simulink model "clik_inverse"  (R2022b)
settings: Solver=ode1  StartTime=0.0  StopTime=4  FixedStep=0.001  RelTol=1e-3
undefined symbols (not defined in the file or in its folder): DiscIntNeverNeededParam, q0, Tc
settings Model: Creator=Xp  LastModifiedBy=brigh
settings SolverCC: AlgebraicLoopSolver=TrustRegion
settings DataIOCC: LimitDataPoints=on  SaveFormat=Array  SignalLoggingSaveFormat=ModelDataLogs  ReturnWorkspaceOutputs=off
settings OptimizationCC: ExpressionDepthLimit=2147483647  InitFltsAndDblsToZero=on  LifeSpan=inf
settings DebuggingCC: SaveWithParameterizedLinksMsg=none  UnderspecifiedInitializationDetection=Classic  MergeDetectMultiDrivingBlocksExec=none  SolverPrmCheckMsg=warning  MultiTaskDSMMsg=warning  MultiTaskCondExecSysMsg=none  FcnCallInpInsideContextMsg=warning  UnconnectedInputMsg=warning  UnconnectedOutputMsg=warning  UnconnectedLineMsg=warning  StateNameClashWarn=warning  SFUnexpectedBacktrackingDiag=warning  SFNoUnconditionalDefaultTransitionDiag=warning  SFExecutionAtInitializationDiag=none  SFMachineParentedDataDiag=warning  ArithmeticOperatorsInVariantConditions=warning
settings HardwareCC: ProdBitPerPointer=32  ProdBitPerSizeT=32  ProdBitPerPtrDiffT=32  ProdLargestAtomicFloat=None  ProdIntDivRoundTo=Undefined  ProdEndianess=Unspecified  ProdWordSize=32  ProdHWDeviceType=32-bit Generic
settings ModelReferenceCC: EnableRefExpFcnMdlSchedulingChecks=on  PropagateSignalLabelsOutOfModel=off
settings SFSimCC: CustomCodeUndefinedFunction=UseInterfaceOnly
settings RTWCC: DLArmComputeVersion=19.05
settings CodeAppCC: StateflowObjectComments=on
settings GRTTargetCC: TargetLangStandard=C89/C90 (ANSI)  CombineOutputUpdateFcns=off  GRTInterface=on
settings ConfigComp: CovMetricSettings=dw  CovSaveCumulativeToWorkspaceVar=on  CovSaveSingleToWorkspaceVar=on

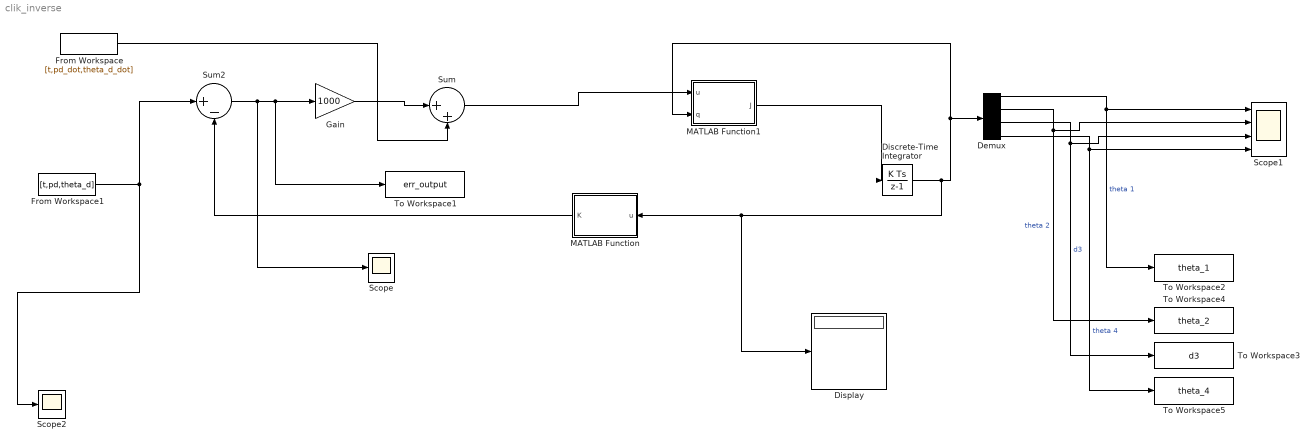
== system clik_inverse ==
  Demux : Demux
  Discrete-Time Integrator : DiscreteIntegrator  InitialCondition=q0  SampleTime=Tc  ICPrevOutput=DiscIntNeverNeededParam  ICPrevScaledInput=DiscIntNeverNeededParam
  Display : Display
  From Workspace : FromWorkspace  VariableName=[t,pd_dot,theta_d_dot]  SampleTime=Tc
  From Workspace1 : FromWorkspace  VariableName=[t,pd,theta_d]  SampleTime=Tc
  Gain : Gain  Gain=1000
  MATLAB Function : MATLAB Function  TreatAsAtomicUnit=on
  MATLAB Function1 : MATLAB Function  TreatAsAtomicUnit=on
  Scope : Scope
  Scope1 : Scope  NumInputPorts=4
  Scope2 : Scope
  Sum : Sum  Inputs=|++
  Sum2 : Sum  Inputs=|+-
  To Workspace1 : ToWorkspace  VariableName=err_output  SampleTime=-1
  To Workspace2 : ToWorkspace  VariableName=theta_1  SampleTime=-1
  To Workspace3 : ToWorkspace  VariableName=d3  SampleTime=-1
  To Workspace4 : ToWorkspace  VariableName=theta_2  SampleTime=-1
  To Workspace5 : ToWorkspace  VariableName=theta_4  SampleTime=-1
  wires:
  From Workspace1/1 -> Scope2/1, Sum2/1
  Sum2/1 -> Scope/1, To Workspace1/1, Gain/1
  Gain/1 -> Sum/1
  Sum/1 -> MATLAB Function1/1(u)
  MATLAB Function1/1(J) -> Discrete-Time Integrator/1
  MATLAB Function/1(K) -> Sum2/2
  From Workspace/1 -> Sum/2
  Demux/1 -> To Workspace2/1, Scope1/1  "theta 1"
  Demux/2 -> To Workspace4/1, Scope1/2  "theta 2"
  Demux/3 -> To Workspace3/1, Scope1/3  "d3"
  Demux/4 -> To Workspace5/1, Scope1/4  "theta 4"
  Discrete-Time Integrator/1 -> Display/1, MATLAB Function/1(u), MATLAB Function1/2(q), Demux/1

== matlab function clik_inverse/MATLAB Function ==
  data: u input; K output
function K = fcn(u)

a1=0.5;
a2=0.5;

theta1=u(1);
theta12 = u(1) + u(2);

cos1 = cos(theta1);
sin1 = sin(theta1);

cos12 = cos(theta12);
sin12 = sin(theta12);

d3=u(3);

K= [a2*cos12+a1*cos1; a2*sin12+a1*sin1; d3; u(1)+u(2)+u(4)];

== matlab function clik_inverse/MATLAB Function1 ==
  data: u input; J output; q input
function J = fcn(u,q)

a1=0.5;
a2= 0.5;


theta1= q(1);
theta12 = q(1)+q(2);

cos1 = cos(theta1);
sin1 = sin(theta1);

cos12 = cos(theta12);
sin12 = sin(theta12);


Jac = [-a2*sin12-a1*sin1 -a2*sin12 0 0; a2*cos12+a1*cos1 a2*cos12 0 0; 0 0 1 0; 1 1 0 1];

J = inv(Jac)* u;
